simulink library "outp"  (Simulink 8.2)
settings: Solver=ode45  SolverMode=SingleTasking  StartTime=0.0  StopTime=10.0  RelTol=1e-3
undefined symbols (not defined in the file or in its folder): EPSILON, KOUTP_ACCSetSpeed_kph_defval, KOUTP_ACCSetSpeed_kph_maxval, KOUTP_ACCSetSpeed_kph_minval, KOUTP_ACCSetSpeed_kph_ovrdflg, KOUTP_ACCSetSpeed_kph_ovrdval, KOUTP_ACCSetSpeed_kph_srvcflg, KOUTP_ACCSetSpeed_kph_srvcval, KOUTP_ACCSetTimeGap_enum_defval, KOUTP_ACCSetTimeGap_enum_ovrdflg, KOUTP_ACCSetTimeGap_enum_ovrdval, KOUTP_ACCSetTimeGap_enum_srvcflg, KOUTP_ACCSetTimeGap_enum_srvcval, KOUTP_ACCSetTimeGapTmp_enum_defval, KOUTP_ACCSetTimeGapTmp_enum_ovrdflg, KOUTP_ACCSetTimeGapTmp_enum_ovrdval, KOUTP_ACCSetTimeGapTmp_enum_srvcflg, KOUTP_ACCSetTimeGapTmp_enum_srvcval, KOUTP_ACCWarningReq_flg_defval, KOUTP_ACCWarningReq_flg_ovrdflg, KOUTP_ACCWarningReq_flg_ovrdval, KOUTP_ACCWarningReq_flg_srvcflg, KOUTP_ACCWarningReq_flg_srvcval, KOUTP_ADAS1RollCnt_cnt_defval, KOUTP_ADAS1RollCnt_cnt_ovrdflg, KOUTP_ADAS1RollCnt_cnt_ovrdval, KOUTP_ADAS1RollCnt_cnt_srvcflg, KOUTP_ADAS1RollCnt_cnt_srvcval, KOUTP_ADAS2RollCnt_cnt_defval, KOUTP_ADAS2RollCnt_cnt_ovrdflg, KOUTP_ADAS2RollCnt_cnt_ovrdval, KOUTP_ADAS2RollCnt_cnt_srvcflg, KOUTP_ADAS2RollCnt_cnt_srvcval, KOUTP_ADAS3RollCnt_cnt_defval, KOUTP_ADAS3RollCnt_cnt_ovrdflg, KOUTP_ADAS3RollCnt_cnt_ovrdval, KOUTP_ADAS3RollCnt_cnt_srvcflg, KOUTP_ADAS3RollCnt_cnt_srvcval, KOUTP_ADASACCStatus_enum_defval, KOUTP_ADASACCStatus_enum_ovrdflg, KOUTP_ADASACCStatus_enum_ovrdval, KOUTP_ADASACCStatus_enum_srvcflg, KOUTP_ADASACCStatus_enum_srvcval, KOUTP_ADASFaultMode_enum_defval, KOUTP_ADASFaultMode_enum_ovrdflg, KOUTP_ADASFaultMode_enum_ovrdval, KOUTP_ADASFaultMode_enum_srvcflg, KOUTP_ADASFaultMode_enum_srvcval, KOUTP_ADASFunOffSoundReq_flg_defval, KOUTP_ADASFunOffSoundReq_flg_ovrdflg, KOUTP_ADASFunOffSoundReq_flg_ovrdval, KOUTP_ADASFunOffSoundReq_flg_srvcflg, KOUTP_ADASFunOffSoundReq_flg_srvcval, KOUTP_ADASFunOnSoundReq_flg_defval, KOUTP_ADASFunOnSoundReq_flg_ovrdflg, KOUTP_ADASFunOnSoundReq_flg_ovrdval, KOUTP_ADASFunOnSoundReq_flg_srvcflg, KOUTP_ADASFunOnSoundReq_flg_srvcval, KOUTP_ADASLFCStatus_enum_defval, KOUTP_ADASLFCStatus_enum_ovrdflg ... (+216)
libraries: outp x52, hcu_lib x8, simulink x3
(part 1 of 2)
settings Model: Creator=WX  LastModifiedBy=14014

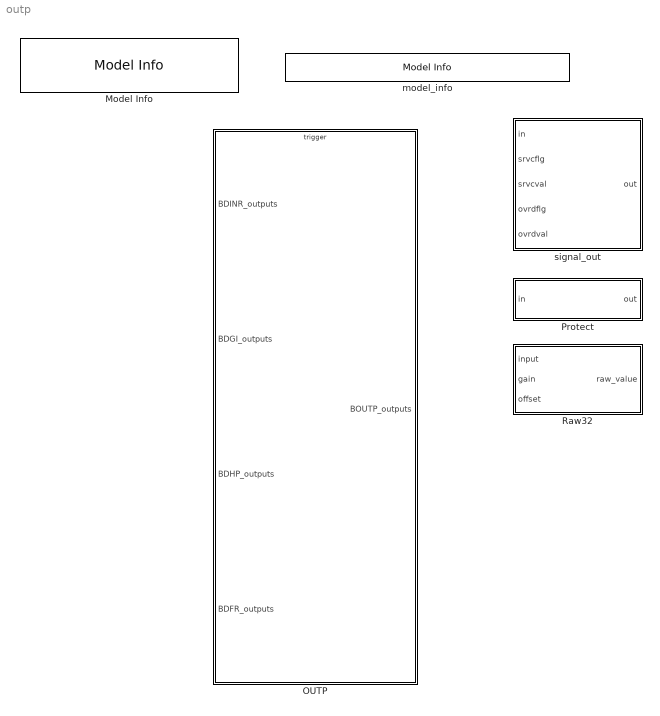
== system outp ==
  Model Info : simulink/Model-Wide Utilities/Model Info  InitialBlockCM=None  BlockCM=None  Frame=on  DisplayStringWithTags=|  HorizontalTextAlignment=Left  LeftAlignmentValue=0.02  SourceBlockDiagram=outp  TagMaxNumber=20
      | Model Version        : %<ModelVersion>
      | Creator                   : %<Creator>
      | Last Modified by    : %<LastModifiedBy>
  OUTP : Subsystem  TreatAsAtomicUnit=on
      settings: RTWSystemCode=Nonreusable function  RTWFcnNameOpts=Use subsystem name  RTWFileNameOpts=Use subsystem name
  Protect : Subsystem
  Raw32 : Subsystem
  model_info : simulink/Model-Wide Utilities/Model Info  InitialBlockCM=None  BlockCM=None  Frame=on  DisplayStringWithTags=$Id: hcu_lib.mdl 289 2016-04-11 06:01:08Z chimotsai $  HorizontalTextAlignment=Center  LeftAlignmentValue=0.5  SourceBlockDiagram=outp  TagMaxNumber=20
  signal_out : Subsystem

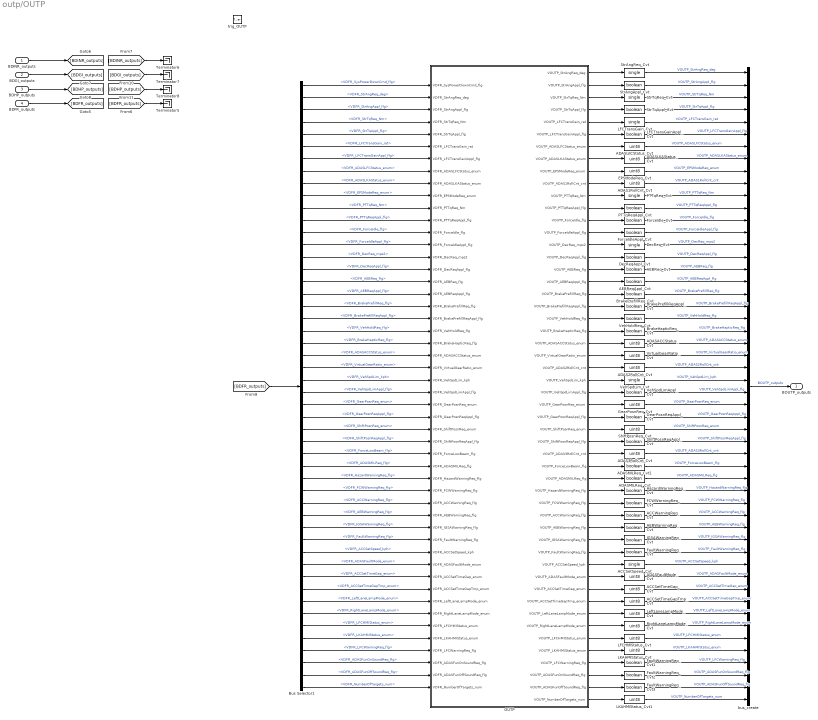
== system outp/OUTP ==
  BDINR_outputs : Inport  OutDataTypeStr=Bus: BDINR_outputs
  BDGI_outputs : Inport  Port=2  OutDataTypeStr=Bus: BDGI_outputs
  BDHP_outputs : Inport  Port=3  OutDataTypeStr=Bus: BDHP_outputs
  BDFR_outputs : Inport  Port=4  OutDataTypeStr=Bus: BDFR_outputs
  trig_OUTP : TriggerPort  TriggerType=function-call
  ACCSetSpeed_Cvt : DataTypeConversion  OutDataTypeStr=single  SaturateOnIntegerOverflow=on  RndMeth=Zero
  ACCSetTimeGapTmp_Cvt : DataTypeConversion  OutDataTypeStr=uint8  SaturateOnIntegerOverflow=on  RndMeth=Zero
  ACCSetTimeGap_Cvt : DataTypeConversion  OutDataTypeStr=uint8  SaturateOnIntegerOverflow=on  RndMeth=Zero
  ACCWarningReq_Cvt : DataTypeConversion  OutDataTypeStr=boolean  SaturateOnIntegerOverflow=on  RndMeth=Zero
  ADAS1RollCnt_Cvt : DataTypeConversion  OutDataTypeStr=uint8  SaturateOnIntegerOverflow=on  RndMeth=Zero
  ADAS2RollCnt_Cvt : DataTypeConversion  OutDataTypeStr=uint8  SaturateOnIntegerOverflow=on  RndMeth=Zero
  ADAS3RollCnt_Cvt : DataTypeConversion  OutDataTypeStr=uint8  SaturateOnIntegerOverflow=on  RndMeth=Zero
  ADASACCStatus_Cvt : DataTypeConversion  OutDataTypeStr=uint8  SaturateOnIntegerOverflow=on  RndMeth=Zero
  ADASFaultMode_Cvt : DataTypeConversion  OutDataTypeStr=uint8  SaturateOnIntegerOverflow=on  RndMeth=Zero
  ADASLFCStatus_Cvt : DataTypeConversion  OutDataTypeStr=uint8  SaturateOnIntegerOverflow=on  RndMeth=Zero
  ADASLKAStatus_Cvt : DataTypeConversion  OutDataTypeStr=uint8  SaturateOnIntegerOverflow=on  RndMeth=Zero
  ADASMILReq_Cvt : DataTypeConversion  OutDataTypeStr=boolean  SaturateOnIntegerOverflow=on  RndMeth=Zero
  ADASMILReq_Cvt1 : DataTypeConversion  OutDataTypeStr=boolean  SaturateOnIntegerOverflow=on  RndMeth=Zero
  AEBReqAppl_Cvt : DataTypeConversion  OutDataTypeStr=boolean  SaturateOnIntegerOverflow=on  RndMeth=Zero
  AEBReq_Cvt : DataTypeConversion  OutDataTypeStr=boolean  SaturateOnIntegerOverflow=on  RndMeth=Zero
  AEBWarningReq_Cvt : DataTypeConversion  OutDataTypeStr=boolean  SaturateOnIntegerOverflow=on  RndMeth=Zero
  BrakeHapticReq_Cvt : DataTypeConversion  OutDataTypeStr=boolean  SaturateOnIntegerOverflow=on  RndMeth=Zero
  BrakePrefillReqAppl_Cvt : DataTypeConversion  OutDataTypeStr=boolean  SaturateOnIntegerOverflow=on  RndMeth=Zero
  BrakePrefillReq_Cvt : DataTypeConversion  OutDataTypeStr=boolean  SaturateOnIntegerOverflow=on  RndMeth=Zero
  Bus Selector1 : BusSelector  OutputSignals=VDFR_SysPowerDownCmd_flg,VDFR_StrAngReq_deg,VDFR_StrAngAppl_flg,VDFR_StrTqReq_Nm,VDFR_StrTqAppl_flg,VDFR_LFCTransGain_rat,VDFR_LFCTransGainAppl_flg,VDFR_ADASLFCStatus_enum,VDFR_ADASLKAStatus_enum,VDFR_EPSModeReq_enum,VDFR_PTTqReq_Nm,VDFR_PTTqReqAppl_flg,VDFR_ForceIdle_flg,VDFR_ForceIdleAppl_flg,VDFR_DecReq_mps2,VDFR_DecReqAppl_flg,VDFR_AEBReq_flg,VDFR_AEBReqAppl_flg,VDFR_BrakePrefillReq_flg,VDFR_BrakePrefillReqAppl_flg,VDFR_VehHoldReq_flg,VDFR_BrakeHapticReq_flg,VDFR_ADASACCStatus_enum,VDFR_VirtualGearRatio_enum,VDFR_VehSpdLim_kph,VDFR_VehSpdLimAppl_flg,VDFR_GearPosnReq_enum,VDFR_GearPosnReqAppl_flg,VDFR_ShiftPosnReq_enum,VDFR_ShiftPosnReqAppl_flg,VDFR_ForceLowBeam_flg,VDFR_ADASMILReq_flg,VDFR_HazardWarningReq_flg,VDFR_FCWWarningReq_flg,VDFR_ACCWarningReq_flg,VDFR_AEBWarningReq_flg,VDFR_IGSAWarningReq_flg,VDFR_FaultWarningReq_flg,VDFR_ACCSetSpeed_kph,VDFR_ADASFaultMode_enum,VDFR_ACCSetTimeGap_enum,VDFR_ACCSetTimeGapTmp_enum,VDFR_LeftLaneLampMode_enum,VDFR_RightLaneLampMode_enum,VDFR_LFCHMIStatus_enum,VDFR_LKAHMIStatus_enum,VDFR_LFCWarningReq_flg,VDFR_ADASFunOnSoundReq_flg,VDFR_ADASFunOffSoundReq_flg,VDFR_NumberOfTargets_num
  DecReqAppl_Cvt : DataTypeConversion  OutDataTypeStr=boolean  SaturateOnIntegerOverflow=on  RndMeth=Zero
  DecReq_Cvt : DataTypeConversion  OutDataTypeStr=single  SaturateOnIntegerOverflow=on  RndMeth=Zero
  EPSModeReq_Cvt : DataTypeConversion  OutDataTypeStr=uint8  SaturateOnIntegerOverflow=on  RndMeth=Zero
  FCWWarningReq_Cvt : DataTypeConversion  OutDataTypeStr=boolean  SaturateOnIntegerOverflow=on  RndMeth=Zero
  FaultWarningReq_Cvt{,1..3} (4 alike) : DataTypeConversion  OutDataTypeStr=boolean  SaturateOnIntegerOverflow=on  RndMeth=Zero
  ForceIdleAppl_Cvt : DataTypeConversion  OutDataTypeStr=boolean  SaturateOnIntegerOverflow=on  RndMeth=Zero
  ForceIdle_Cvt : DataTypeConversion  OutDataTypeStr=boolean  SaturateOnIntegerOverflow=on  RndMeth=Zero
  GearPosnReqAppl_Cvt : DataTypeConversion  OutDataTypeStr=boolean  SaturateOnIntegerOverflow=on  RndMeth=Zero
  GearPosnReq_Cvt : DataTypeConversion  OutDataTypeStr=uint8  SaturateOnIntegerOverflow=on  RndMeth=Zero
  HazardWarningReq_Cvt : DataTypeConversion  OutDataTypeStr=boolean  SaturateOnIntegerOverflow=on  RndMeth=Zero
  IGSAWarningReq_Cvt : DataTypeConversion  OutDataTypeStr=boolean  SaturateOnIntegerOverflow=on  RndMeth=Zero
  LFCHMIStatus_Cvt : DataTypeConversion  OutDataTypeStr=uint8  SaturateOnIntegerOverflow=on  RndMeth=Zero
  LFCTransGainAppl_Cvt : DataTypeConversion  OutDataTypeStr=boolean  SaturateOnIntegerOverflow=on  RndMeth=Zero
  LFCTransGain_Cvt : DataTypeConversion  OutDataTypeStr=single  SaturateOnIntegerOverflow=on  RndMeth=Zero
  LKAHMIStatus_Cvt : DataTypeConversion  OutDataTypeStr=uint8  SaturateOnIntegerOverflow=on  RndMeth=Zero
  LKAHMIStatus_Cvt1 : DataTypeConversion  OutDataTypeStr=uint8  SaturateOnIntegerOverflow=on  RndMeth=Zero
  LeftLaneLampMode_Cvt : DataTypeConversion  OutDataTypeStr=uint8  SaturateOnIntegerOverflow=on  RndMeth=Zero
  OUTP : Subsystem
  PTTqReqAppl_Cvt : DataTypeConversion  OutDataTypeStr=boolean  SaturateOnIntegerOverflow=on  RndMeth=Zero
  PTTqReq_Cvt : DataTypeConversion  OutDataTypeStr=single  SaturateOnIntegerOverflow=on  RndMeth=Zero
  RightLaneLampMode_Cvt : DataTypeConversion  OutDataTypeStr=uint8  SaturateOnIntegerOverflow=on  RndMeth=Zero
  ShiftPosnReqAppl_Cvt : DataTypeConversion  OutDataTypeStr=boolean  SaturateOnIntegerOverflow=on  RndMeth=Zero
  ShiftPosnReq_Cvt : DataTypeConversion  OutDataTypeStr=uint8  SaturateOnIntegerOverflow=on  RndMeth=Zero
  StrAngAppl_Cvt : DataTypeConversion  OutDataTypeStr=boolean  SaturateOnIntegerOverflow=on  RndMeth=Zero
  StrAngReq_Cvt : DataTypeConversion  OutDataTypeStr=single  SaturateOnIntegerOverflow=on  RndMeth=Zero
  StrTqAppl_Cvt : DataTypeConversion  OutDataTypeStr=boolean  SaturateOnIntegerOverflow=on  RndMeth=Zero
  StrTqReq_Cvt : DataTypeConversion  OutDataTypeStr=single  SaturateOnIntegerOverflow=on  RndMeth=Zero
  Terminator{5..8} (4 alike) : Terminator
  VehHoldReq_Cvt : DataTypeConversion  OutDataTypeStr=boolean  SaturateOnIntegerOverflow=on  RndMeth=Zero
  VehSpdLimAppl_Cvt : DataTypeConversion  OutDataTypeStr=boolean  SaturateOnIntegerOverflow=on  RndMeth=Zero
  VehSpdLim_Cvt : DataTypeConversion  OutDataTypeStr=single  SaturateOnIntegerOverflow=on  RndMeth=Zero
  VirtualGearRatio_Cvt : DataTypeConversion  OutDataTypeStr=uint8  SaturateOnIntegerOverflow=on  RndMeth=Zero
  bus_create : BusCreator  Inputs=52  OutDataTypeStr=Bus: BOUTP_outputs
  BOUTP_outputs : Outport  OutDataTypeStr=Bus: BOUTP_outputs
  wires:
  [BDFR_outputs] -> Bus Selector1/1
  [BDFR_outputs] -> Terminator5/1
  BDFR_outputs/1 -> [BDFR_outputs]
  [BDINR_outputs] -> Terminator6/1
  BDINR_outputs/1 -> [BDINR_outputs]
  [BDGI_outputs] -> Terminator7/1
  BDGI_outputs/1 -> [BDGI_outputs]
  [BDHP_outputs] -> Terminator8/1
  BDHP_outputs/1 -> [BDHP_outputs]
  bus_create/1 -> BOUTP_outputs/1  "BOUTP_outputs"
  StrAngReq_Cvt/1 -> bus_create/1  "VOUTP_StrAngReq_deg"
  StrAngAppl_Cvt/1 -> bus_create/2  "VOUTP_StrAngAppl_flg"
  StrTqReq_Cvt/1 -> bus_create/3  "VOUTP_StrTqReq_Nm"
  StrTqAppl_Cvt/1 -> bus_create/4  "VOUTP_StrTqAppl_flg"
  LFCTransGain_Cvt/1 -> bus_create/5  "VOUTP_LFCTransGain_rat"
  LFCTransGainAppl_Cvt/1 -> bus_create/6  "VOUTP_LFCTransGainAppl_flg"
  ADASLFCStatus_Cvt/1 -> bus_create/7  "VOUTP_ADASLFCStatus_enum"
  ADASLKAStatus_Cvt/1 -> bus_create/8  "VOUTP_ADASLKAStatus_enum"
  EPSModeReq_Cvt/1 -> bus_create/9  "VOUTP_EPSModeReq_enum"
  ADAS1RollCnt_Cvt/1 -> bus_create/10  "VOUTP_ADAS1RollCnt_cnt"
  PTTqReq_Cvt/1 -> bus_create/11  "VOUTP_PTTqReq_Nm"
  ForceIdle_Cvt/1 -> bus_create/13  "VOUTP_ForceIdle_flg"
  PTTqReqAppl_Cvt/1 -> bus_create/12  "VOUTP_PTTqReqAppl_flg"
  DecReqAppl_Cvt/1 -> bus_create/16  "VOUTP_DecReqAppl_flg"
  ForceIdleAppl_Cvt/1 -> bus_create/14  "VOUTP_ForceIdleAppl_flg"
  DecReq_Cvt/1 -> bus_create/15  "VOUTP_DecReq_mps2"
  AEBReq_Cvt/1 -> bus_create/17  "VOUTP_AEBReq_flg"
  AEBReqAppl_Cvt/1 -> bus_create/18  "VOUTP_AEBReqAppl_flg"
  BrakePrefillReq_Cvt/1 -> bus_create/19  "VOUTP_BrakePrefillReq_flg"
  BrakePrefillReqAppl_Cvt/1 -> bus_create/20  "VOUTP_BrakePrefillReqAppl_flg"
  VehHoldReq_Cvt/1 -> bus_create/21  "VOUTP_VehHoldReq_flg"
  BrakeHapticReq_Cvt/1 -> bus_create/22  "VOUTP_BrakeHapticReq_flg"
  ADASACCStatus_Cvt/1 -> bus_create/23  "VOUTP_ADASACCStatus_enum"
  VirtualGearRatio_Cvt/1 -> bus_create/24  "VOUTP_VirtualGearRatio_enum"
  ADAS2RollCnt_Cvt/1 -> bus_create/25  "VOUTP_ADAS2RollCnt_cnt"
  VehSpdLim_Cvt/1 -> bus_create/26  "VOUTP_VehSpdLim_kph"
  VehSpdLimAppl_Cvt/1 -> bus_create/27  "VOUTP_VehSpdLimAppl_flg"
  GearPosnReq_Cvt/1 -> bus_create/28  "VOUTP_GearPosnReq_enum"
  GearPosnReqAppl_Cvt/1 -> bus_create/29  "VOUTP_GearPosnReqAppl_flg"
  ShiftPosnReq_Cvt/1 -> bus_create/30  "VOUTP_ShiftPosnReq_enum"
  ShiftPosnReqAppl_Cvt/1 -> bus_create/31  "VOUTP_ShiftPosnReqAppl_flg"
  ADAS3RollCnt_Cvt/1 -> bus_create/32  "VOUTP_ADAS3RollCnt_cnt"
  ADASMILReq_Cvt/1 -> bus_create/34  "VOUTP_ADASMILReq_flg"
  HazardWarningReq_Cvt/1 -> bus_create/35  "VOUTP_HazardWarningReq_flg"
  FCWWarningReq_Cvt/1 -> bus_create/36  "VOUTP_FCWWarningReq_flg"
  ACCWarningReq_Cvt/1 -> bus_create/37  "VOUTP_ACCWarningReq_flg"
  AEBWarningReq_Cvt/1 -> bus_create/38  "VOUTP_AEBWarningReq_flg"
  IGSAWarningReq_Cvt/1 -> bus_create/39  "VOUTP_IGSAWarningReq_flg"
  FaultWarningReq_Cvt/1 -> bus_create/40  "VOUTP_FaultWarningReq_flg"
  ACCSetSpeed_Cvt/1 -> bus_create/41  "VOUTP_ACCSetSpeed_kph"
  ADASFaultMode_Cvt/1 -> bus_create/42  "VOUTP_ADASFaultMode_enum"
  ACCSetTimeGap_Cvt/1 -> bus_create/43  "VOUTP_ACCSetTimeGap_enum"
  ACCSetTimeGapTmp_Cvt/1 -> bus_create/44  "VOUTP_ACCSetTimeGapTmp_enum"
  LeftLaneLampMode_Cvt/1 -> bus_create/45  "VOUTP_LeftLaneLampMode_enum"
  RightLaneLampMode_Cvt/1 -> bus_create/46  "VOUTP_RightLaneLampMode_enum"
  LFCHMIStatus_Cvt/1 -> bus_create/47  "VOUTP_LFCHMIStatus_enum"
  LKAHMIStatus_Cvt/1 -> bus_create/48  "VOUTP_LKAHMIStatus_enum"
  ADASMILReq_Cvt1/1 -> bus_create/33  "VOUTP_ForceLowBeam_flg"
  OUTP/30(VOUTP_ShiftPosnReq_enum) -> ShiftPosnReq_Cvt/1
  OUTP/14(VOUTP_ForceIdleAppl_flg) -> ForceIdleAppl_Cvt/1
  OUTP/4(VOUTP_StrTqAppl_flg) -> StrTqAppl_Cvt/1
  OUTP/13(VOUTP_ForceIdle_flg) -> ForceIdle_Cvt/1
  OUTP/29(VOUTP_GearPosnReqAppl_flg) -> GearPosnReqAppl_Cvt/1
  OUTP/27(VOUTP_VehSpdLimAppl_flg) -> VehSpdLimAppl_Cvt/1
  OUTP/2(VOUTP_StrAngAppl_flg) -> StrAngAppl_Cvt/1
  OUTP/26(VOUTP_VehSpdLim_kph) -> VehSpdLim_Cvt/1
  OUTP/6(VOUTP_LFCTransGainAppl_flg) -> LFCTransGainAppl_Cvt/1
  OUTP/10(VOUTP_ADAS1RollCnt_cnt) -> ADAS1RollCnt_Cvt/1
  OUTP/35(VOUTP_HazardWarningReq_flg) -> HazardWarningReq_Cvt/1
  OUTP/18(VOUTP_AEBReqAppl_flg) -> AEBReqAppl_Cvt/1
  OUTP/38(VOUTP_AEBWarningReq_flg) -> AEBWarningReq_Cvt/1
  OUTP/43(VOUTP_ACCSetTimeGap_enum) -> ACCSetTimeGap_Cvt/1
  OUTP/41(VOUTP_ACCSetSpeed_kph) -> ACCSetSpeed_Cvt/1
  OUTP/31(VOUTP_ShiftPosnReqAppl_flg) -> ShiftPosnReqAppl_Cvt/1
  OUTP/8(VOUTP_ADASLKAStatus_enum) -> ADASLKAStatus_Cvt/1
  OUTP/44(VOUTP_ACCSetTimeGapTmp_enum) -> ACCSetTimeGapTmp_Cvt/1
  OUTP/47(VOUTP_LFCHMIStatus_enum) -> LFCHMIStatus_Cvt/1
  OUTP/17(VOUTP_AEBReq_flg) -> AEBReq_Cvt/1
  OUTP/34(VOUTP_ADASMILReq_flg) -> ADASMILReq_Cvt/1
  OUTP/16(VOUTP_DecReqAppl_flg) -> DecReqAppl_Cvt/1
  OUTP/5(VOUTP_LFCTransGain_rat) -> LFCTransGain_Cvt/1
  OUTP/32(VOUTP_ADAS3RollCnt_cnt) -> ADAS3RollCnt_Cvt/1
  OUTP/12(VOUTP_PTTqReqAppl_flg) -> PTTqReqAppl_Cvt/1
  OUTP/9(VOUTP_EPSModeReq_enum) -> EPSModeReq_Cvt/1
  OUTP/7(VOUTP_ADASLFCStatus_enum) -> ADASLFCStatus_Cvt/1
  OUTP/42(VOUTP_ADASFaultMode_enum) -> ADASFaultMode_Cvt/1
  OUTP/11(VOUTP_PTTqReq_Nm) -> PTTqReq_Cvt/1
  OUTP/3(VOUTP_StrTqReq_Nm) -> StrTqReq_Cvt/1
  OUTP/40(VOUTP_FaultWarningReq_flg) -> FaultWarningReq_Cvt/1
  OUTP/25(VOUTP_ADAS2RollCnt_cnt) -> ADAS2RollCnt_Cvt/1
  OUTP/36(VOUTP_FCWWarningReq_flg) -> FCWWarningReq_Cvt/1
  OUTP/48(VOUTP_LKAHMIStatus_enum) -> LKAHMIStatus_Cvt/1
  OUTP/22(VOUTP_BrakeHapticReq_flg) -> BrakeHapticReq_Cvt/1
  OUTP/37(VOUTP_ACCWarningReq_flg) -> ACCWarningReq_Cvt/1
  OUTP/46(VOUTP_RightLaneLampMode_enum) -> RightLaneLampMode_Cvt/1
  OUTP/15(VOUTP_DecReq_mps2) -> DecReq_Cvt/1
  OUTP/23(VOUTP_ADASACCStatus_enum) -> ADASACCStatus_Cvt/1
  OUTP/45(VOUTP_LeftLaneLampMode_enum) -> LeftLaneLampMode_Cvt/1
  OUTP/28(VOUTP_GearPosnReq_enum) -> GearPosnReq_Cvt/1
  OUTP/20(VOUTP_BrakePrefillReqAppl_flg) -> BrakePrefillReqAppl_Cvt/1
  OUTP/39(VOUTP_IGSAWarningReq_flg) -> IGSAWarningReq_Cvt/1
  OUTP/19(VOUTP_BrakePrefillReq_flg) -> BrakePrefillReq_Cvt/1
  OUTP/21(VOUTP_VehHoldReq_flg) -> VehHoldReq_Cvt/1
  OUTP/1(VOUTP_StrAngReq_deg) -> StrAngReq_Cvt/1
  OUTP/24(VOUTP_VirtualGearRatio_enum) -> VirtualGearRatio_Cvt/1
  OUTP/33(VOUTP_ForceLowBeam_flg) -> ADASMILReq_Cvt1/1
  Bus Selector1/7 -> OUTP/7(VDFR_LFCTransGainAppl_flg)  "<VDFR_LFCTransGainAppl_flg>"
  Bus Selector1/8 -> OUTP/8(VDFR_ADASLFCStatus_enum)  "<VDFR_ADASLFCStatus_enum>"
  Bus Selector1/9 -> OUTP/9(VDFR_ADASLKAStatus_enum)  "<VDFR_ADASLKAStatus_enum>"
  Bus Selector1/10 -> OUTP/10(VDFR_EPSModeReq_enum)  "<VDFR_EPSModeReq_enum>"
  Bus Selector1/11 -> OUTP/11(VDFR_PTTqReq_Nm)  "<VDFR_PTTqReq_Nm>"
  Bus Selector1/12 -> OUTP/12(VDFR_PTTqReqAppl_flg)  "<VDFR_PTTqReqAppl_flg>"
  Bus Selector1/13 -> OUTP/13(VDFR_ForceIdle_flg)  "<VDFR_ForceIdle_flg>"
  Bus Selector1/14 -> OUTP/14(VDFR_ForceIdleAppl_flg)  "<VDFR_ForceIdleAppl_flg>"
  Bus Selector1/16 -> OUTP/16(VDFR_DecReqAppl_flg)  "<VDFR_DecReqAppl_flg>"
  Bus Selector1/15 -> OUTP/15(VDFR_DecReq_mps2)  "<VDFR_DecReq_mps2>"
  Bus Selector1/17 -> OUTP/17(VDFR_AEBReq_flg)  "<VDFR_AEBReq_flg>"
  Bus Selector1/18 -> OUTP/18(VDFR_AEBReqAppl_flg)  "<VDFR_AEBReqAppl_flg>"
  Bus Selector1/6 -> OUTP/6(VDFR_LFCTransGain_rat)  "<VDFR_LFCTransGain_rat>"
  Bus Selector1/5 -> OUTP/5(VDFR_StrTqAppl_flg)  "<VDFR_StrTqAppl_flg>"
  Bus Selector1/19 -> OUTP/19(VDFR_BrakePrefillReq_flg)  "<VDFR_BrakePrefillReq_flg>"
  Bus Selector1/1 -> OUTP/1(VDFR_SysPowerDownCmd_flg)  "<VDFR_SysPowerDownCmd_flg>"
  Bus Selector1/4 -> OUTP/4(VDFR_StrTqReq_Nm)  "<VDFR_StrTqReq_Nm>"
  Bus Selector1/3 -> OUTP/3(VDFR_StrAngAppl_flg)  "<VDFR_StrAngAppl_flg>"
  Bus Selector1/2 -> OUTP/2(VDFR_StrAngReq_deg)  "<VDFR_StrAngReq_deg>"
  Bus Selector1/21 -> OUTP/21(VDFR_VehHoldReq_flg)  "<VDFR_VehHoldReq_flg>"
  Bus Selector1/20 -> OUTP/20(VDFR_BrakePrefillReqAppl_flg)  "<VDFR_BrakePrefillReqAppl_flg>"
  Bus Selector1/22 -> OUTP/22(VDFR_BrakeHapticReq_flg)  "<VDFR_BrakeHapticReq_flg>"
  Bus Selector1/23 -> OUTP/23(VDFR_ADASACCStatus_enum)  "<VDFR_ADASACCStatus_enum>"
  Bus Selector1/35 -> OUTP/35(VDFR_ACCWarningReq_flg)  "<VDFR_ACCWarningReq_flg>"
  Bus Selector1/37 -> OUTP/37(VDFR_IGSAWarningReq_flg)  "<VDFR_IGSAWarningReq_flg>"
  Bus Selector1/28 -> OUTP/28(VDFR_GearPosnReqAppl_flg)  "<VDFR_GearPosnReqAppl_flg>"
  Bus Selector1/26 -> OUTP/26(VDFR_VehSpdLimAppl_flg)  "<VDFR_VehSpdLimAppl_flg>"
  Bus Selector1/31 -> OUTP/31(VDFR_ForceLowBeam_flg)  "<VDFR_ForceLowBeam_flg>"
  Bus Selector1/24 -> OUTP/24(VDFR_VirtualGearRatio_enum)  "<VDFR_VirtualGearRatio_enum>"
  Bus Selector1/33 -> OUTP/33(VDFR_HazardWarningReq_flg)  "<VDFR_HazardWarningReq_flg>"
  Bus Selector1/41 -> OUTP/41(VDFR_ACCSetTimeGap_enum)  "<VDFR_ACCSetTimeGap_enum>"
  Bus Selector1/34 -> OUTP/34(VDFR_FCWWarningReq_flg)  "<VDFR_FCWWarningReq_flg>"
  Bus Selector1/43 -> OUTP/43(VDFR_LeftLaneLampMode_enum)  "<VDFR_LeftLaneLampMode_enum>"
  Bus Selector1/30 -> OUTP/30(VDFR_ShiftPosnReqAppl_flg)  "<VDFR_ShiftPosnReqAppl_flg>"
  Bus Selector1/40 -> OUTP/40(VDFR_ADASFaultMode_enum)  "<VDFR_ADASFaultMode_enum>"
  Bus Selector1/38 -> OUTP/38(VDFR_FaultWarningReq_flg)  "<VDFR_FaultWarningReq_flg>"
  Bus Selector1/36 -> OUTP/36(VDFR_AEBWarningReq_flg)  "<VDFR_AEBWarningReq_flg>"
  Bus Selector1/29 -> OUTP/29(VDFR_ShiftPosnReq_enum)  "<VDFR_ShiftPosnReq_enum>"
  Bus Selector1/46 -> OUTP/46(VDFR_LKAHMIStatus_enum)  "<VDFR_LKAHMIStatus_enum>"
  Bus Selector1/27 -> OUTP/27(VDFR_GearPosnReq_enum)  "<VDFR_GearPosnReq_enum>"
  Bus Selector1/32 -> OUTP/32(VDFR_ADASMILReq_flg)  "<VDFR_ADASMILReq_flg>"
  Bus Selector1/45 -> OUTP/45(VDFR_LFCHMIStatus_enum)  "<VDFR_LFCHMIStatus_enum>"
  Bus Selector1/25 -> OUTP/25(VDFR_VehSpdLim_kph)  "<VDFR_VehSpdLim_kph>"
  Bus Selector1/44 -> OUTP/44(VDFR_RightLaneLampMode_enum)  "<VDFR_RightLaneLampMode_enum>"
  Bus Selector1/39 -> OUTP/39(VDFR_ACCSetSpeed_kph)  "<VDFR_ACCSetSpeed_kph>"
  Bus Selector1/42 -> OUTP/42(VDFR_ACCSetTimeGapTmp_enum)  "<VDFR_ACCSetTimeGapTmp_enum>"
  Bus Selector1/48 -> OUTP/48(VDFR_ADASFunOnSoundReq_flg)  "<VDFR_ADASFunOnSoundReq_flg>"
  Bus Selector1/47 -> OUTP/47(VDFR_LFCWarningReq_flg)  "<VDFR_LFCWarningReq_flg>"
  Bus Selector1/50 -> OUTP/50(VDFR_NumberOfTargets_num)  "<VDFR_NumberOfTargets_num>"
  Bus Selector1/49 -> OUTP/49(VDFR_ADASFunOffSoundReq_flg)  "<VDFR_ADASFunOffSoundReq_flg>"
  OUTP/49(VOUTP_LFCWarningReq_flg) -> FaultWarningReq_Cvt1/1
  OUTP/50(VOUTP_ADASFunOnSoundReq_flg) -> FaultWarningReq_Cvt2/1
  OUTP/51(VOUTP_ADASFunOffSoundReq_flg) -> FaultWarningReq_Cvt3/1
  OUTP/52(VOUTP_NumberOfTargets_num) -> LKAHMIStatus_Cvt1/1
  LKAHMIStatus_Cvt1/1 -> bus_create/52  "VOUTP_NumberOfTargets_num"
  FaultWarningReq_Cvt3/1 -> bus_create/51  "VOUTP_ADASFunOffSoundReq_flg"
  FaultWarningReq_Cvt1/1 -> bus_create/49  "VOUTP_LFCWarningReq_flg"
  FaultWarningReq_Cvt2/1 -> bus_create/50  "VOUTP_ADASFunOnSoundReq_flg"

== system outp/Protect ==
  in : Inport
  Bias : Bias  Bias=1
  Bitwise Operator : simulink/Logic and Bit Operations/Bitwise Operator  logicop=NOT  UseBitMask=off  BitMask=bin2dec('11011001')  BitMaskRealWorld=Stored Integer
  out : Outport
  wires:
  Bitwise Operator/1 -> Bias/1
  Bias/1 -> out/1
  in/1 -> Bitwise Operator/1

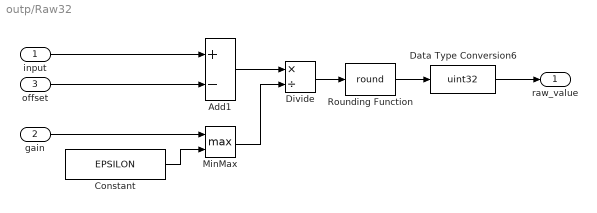
== system outp/Raw32 ==
  input : Inport
  gain : Inport  Port=2
  offset : Inport  Port=3
  Add1 : Sum  Inputs=+-
  Constant : Constant  Value=EPSILON
  Data Type Conversion6 : DataTypeConversion  OutDataTypeStr=uint32
  Divide : Product  Inputs=*/
  MinMax : MinMax  Function=max  Inputs=2
  Rounding Function : Rounding  Operator=round
  raw_value : Outport
  wires:
  Data Type Conversion6/1 -> raw_value/1
  Rounding Function/1 -> Data Type Conversion6/1
  input/1 -> Add1/1
  offset/1 -> Add1/2
  Add1/1 -> Divide/1
  Divide/1 -> Rounding Function/1
  gain/1 -> MinMax/1
  MinMax/1 -> Divide/2
  Constant/1 -> MinMax/2

== system outp/signal_out ==
  in : Inport
  srvcflg : Inport  Port=2
  srvcval : Inport  Port=3
  ovrdflg : Inport  Port=4
  ovrdval : Inport  Port=5
  Constant1 : Constant  Value=TRUE  OutDataTypeStr=Inherit: Inherit via back propagation
  Terminator13 : Terminator
  override signal : hcu_lib/override signal
  out : Outport
  wires:
  in/1 -> override signal/2
  override signal/1 -> out/1
  Constant1/1 -> override signal/1
  srvcflg/1 -> override signal/3
  srvcval/1 -> override signal/4
  ovrdflg/1 -> override signal/5
  ovrdval/1 -> override signal/6
  override signal/2 -> Terminator13/1

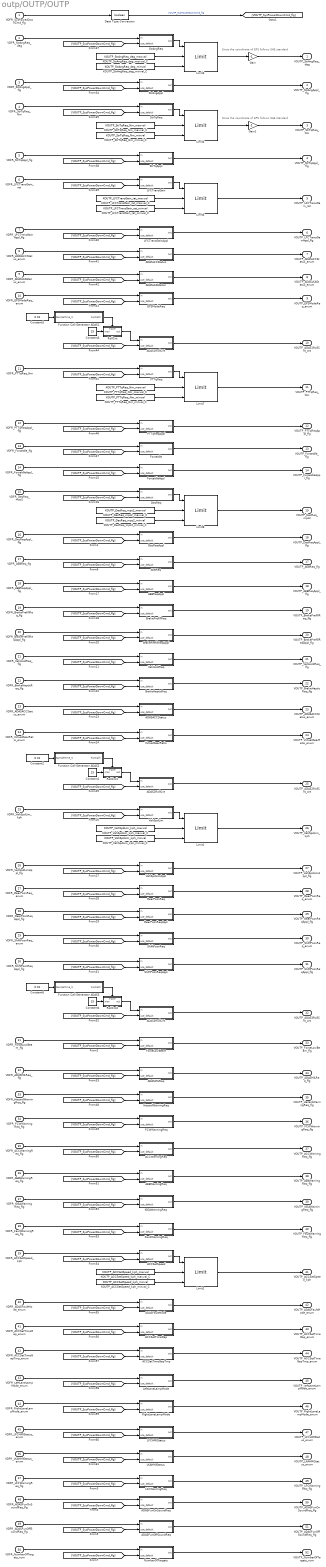
== system outp/OUTP/OUTP ==
  note: Since the coordinate of EPS follows SAE standard
  note: Since the coordinate of EPS follows SAE standard
  VDFR_SysPowerDownCmd_flg : Inport
  VDFR_StrAngReq_deg : Inport  Port=2
  VDFR_StrAngAppl_flg : Inport  Port=3
  VDFR_StrTqReq_Nm : Inport  Port=4
  VDFR_StrTqAppl_flg : Inport  Port=5
  VDFR_LFCTransGain_rat : Inport  Port=6
  VDFR_LFCTransGainAppl_flg : Inport  Port=7
  VDFR_ADASLFCStatus_enum : Inport  Port=8
  VDFR_ADASLKAStatus_enum : Inport  Port=9
  VDFR_EPSModeReq_enum : Inport  Port=10
  VDFR_PTTqReq_Nm : Inport  Port=11
  VDFR_PTTqReqAppl_flg : Inport  Port=12
  VDFR_ForceIdle_flg : Inport  Port=13
  VDFR_ForceIdleAppl_flg : Inport  Port=14
  VDFR_DecReq_mps2 : Inport  Port=15
  VDFR_DecReqAppl_flg : Inport  Port=16
  VDFR_AEBReq_flg : Inport  Port=17
  VDFR_AEBReqAppl_flg : Inport  Port=18
  VDFR_BrakePrefillReq_flg : Inport  Port=19
  VDFR_BrakePrefillReqAppl_flg : Inport  Port=20
  VDFR_VehHoldReq_flg : Inport  Port=21
  VDFR_BrakeHapticReq_flg : Inport  Port=22
  VDFR_ADASACCStatus_enum : Inport  Port=23
  VDFR_VirtualGearRatio_enum : Inport  Port=24
  VDFR_VehSpdLim_kph : Inport  Port=25
  VDFR_VehSpdLimAppl_flg : Inport  Port=26
  VDFR_GearPosnReq_enum : Inport  Port=27
  VDFR_GearPosnReqAppl_flg : Inport  Port=28
  VDFR_ShiftPosnReq_enum : Inport  Port=29
  VDFR_ShiftPosnReqAppl_flg : Inport  Port=30
  VDFR_ForceLowBeam_flg : Inport  Port=31
  VDFR_ADASMILReq_flg : Inport  Port=32
  VDFR_HazardWarningReq_flg : Inport  Port=33
  VDFR_FCWWarningReq_flg : Inport  Port=34
  VDFR_ACCWarningReq_flg : Inport  Port=35
  VDFR_AEBWarningReq_flg : Inport  Port=36
  VDFR_IGSAWarningReq_flg : Inport  Port=37
  VDFR_FaultWarningReq_flg : Inport  Port=38
  VDFR_ACCSetSpeed_kph : Inport  Port=39
  VDFR_ADASFaultMode_enum : Inport  Port=40
  VDFR_ACCSetTimeGap_enum : Inport  Port=41
  VDFR_ACCSetTimeGapTmp_enum : Inport  Port=42
  VDFR_LeftLaneLampMode_enum : Inport  Port=43
  VDFR_RightLaneLampMode_enum : Inport  Port=44
  VDFR_LFCHMIStatus_enum : Inport  Port=45
  VDFR_LKAHMIStatus_enum : Inport  Port=46
  VDFR_LFCWarningReq_flg : Inport  Port=47
  VDFR_ADASFunOnSoundReq_flg : Inport  Port=48
  VDFR_ADASFunOffSoundReq_flg : Inport  Port=49
  VDFR_NumberOfTargets_num : Inport  Port=50
  ACCSetSpeed : Subsystem
  ACCSetTimeGap : Subsystem
  ACCSetTimeGapTmp : Subsystem
  ACCWarningReq : Subsystem
  ADAS1RollCnt : Subsystem
  ADAS2RollCnt : Subsystem
  ADAS3RollCnt : Subsystem
  ADASACCStatus : Subsystem
  ADASFaultMode : Subsystem
  ADASFunOffSoundReq : Subsystem
  ADASFunOnSoundReq : Subsystem
  ADASLFCStatus : Subsystem
  ADASLKAStatus : Subsystem
  ADASMILReq : Subsystem
  AEBReq : Subsystem
  AEBReqAppl : Subsystem
  AEBWarningReq : Subsystem
  BrakeHapticReq : Subsystem
  BrakePrefillReq : Subsystem
  BrakePrefillReqAppl : Subsystem
  Constant1 : Constant  Value=15  OutDataTypeStr=uint8
  Constant2 : Constant  Value=0.01
  Constant3 : Constant  Value=15  OutDataTypeStr=uint8
  Constant4 : Constant  Value=15  OutDataTypeStr=uint8
  Constant5 : Constant  Value=0.01
  Constant6 : Constant  Value=0.01
  Data Type Conversion : DataTypeConversion  OutDataTypeStr=boolean
  DecReq : Subsystem
  DecReqAppl : Subsystem
  EPSModeReq : Subsystem
  FCWWarningReq : Subsystem
  FaultWarningReq : Subsystem
  ForceIdle : Subsystem
  ForceIdleAppl : Subsystem
  ForceLowBeam : Subsystem
  Function Call Generator ADAS1 : Stateflow chart  TreatAsAtomicUnit=on
  Function Call Generator ADAS2 : Stateflow chart  TreatAsAtomicUnit=on
  Function Call Generator ADAS3 : Stateflow chart  TreatAsAtomicUnit=on
  Gain : Gain  Gain=-1
  Gain1 : Gain  Gain=-1
  GearPosnReq : Subsystem
  GearPosnReqAppl : Subsystem
  HazardWarningReq : Subsystem
  IGSAWarningReq : Subsystem
  KOUTP_ACCSetSpeed_kph_maxval_C : Constant  Value=KOUTP_ACCSetSpeed_kph_maxval
  KOUTP_ACCSetSpeed_kph_minval_C : Constant  Value=KOUTP_ACCSetSpeed_kph_minval
  KOUTP_DecReq_mps2_maxval_C : Constant  Value=KOUTP_DecReq_mps2_maxval
  KOUTP_DecReq_mps2_minval_C : Constant  Value=KOUTP_DecReq_mps2_minval
  KOUTP_LFCTransGain_rat_maxval_C : Constant  Value=KOUTP_LFCTransGain_rat_maxval
  KOUTP_LFCTransGain_rat_minval_C : Constant  Value=KOUTP_LFCTransGain_rat_minval
  KOUTP_PTTqReq_Nm_maxval_C : Constant  Value=KOUTP_PTTqReq_Nm_maxval
  KOUTP_PTTqReq_Nm_minval_C : Constant  Value=KOUTP_PTTqReq_Nm_minval
  KOUTP_StrAngReq_deg_maxval_C : Constant  Value=KOUTP_StrAngReq_deg_maxval
  KOUTP_StrAngReq_deg_minval_C : Constant  Value=KOUTP_StrAngReq_deg_minval
  KOUTP_StrTqReq_Nm_maxval_C : Constant  Value=KOUTP_StrTqReq_Nm_maxval
  KOUTP_StrTqReq_Nm_minval_C : Constant  Value=KOUTP_StrTqReq_Nm_minval
  KOUTP_VehSpdLim_kph_maxval_C : Constant  Value=KOUTP_VehSpdLim_kph_maxval
  KOUTP_VehSpdLim_kph_minval_C : Constant  Value=KOUTP_VehSpdLim_kph_minval
  LFCHMIStatus : Subsystem
  LFCTransGain : Subsystem
  LFCTransGainAppl : Subsystem
  LFCWarningReq : Subsystem
  LKAHMIStatus : Subsystem
  LeftLaneLampMode : Subsystem
  Limit{1..4,6..8} (7 alike) : hcu_lib/Limit  SystemSampleTime=-1
  NumberOfTargets : Subsystem
  PTTqReq : Subsystem
  PTTqReqAppl : Subsystem
  RightLaneLampMode : Subsystem
  RollCnt : Subsystem
  RollCnt1 : Subsystem
  RollCnt2 : Subsystem
  ShiftPosnReq : Subsystem
  ShiftPosnReqAppl : Subsystem
  StrAngAppl : Subsystem
  StrAngReq : Subsystem
  StrTqAppl : Subsystem
  StrTqReq : Subsystem
  VehHoldReq : Subsystem
  VehSpdLim : Subsystem
  VehSpdLimAppl : Subsystem
  VirtualGearRatio : Subsystem
  VOUTP_StrAngReq_deg : Outport
  VOUTP_StrAngAppl_flg : Outport  Port=2
  VOUTP_StrTqReq_Nm : Outport  Port=3
  VOUTP_StrTqAppl_flg : Outport  Port=4
  VOUTP_LFCTransGain_rat : Outport  Port=5
  VOUTP_LFCTransGainAppl_flg : Outport  Port=6
  VOUTP_ADASLFCStatus_enum : Outport  Port=7
  VOUTP_ADASLKAStatus_enum : Outport  Port=8
  VOUTP_EPSModeReq_enum : Outport  Port=9
  VOUTP_ADAS1RollCnt_cnt : Outport  Port=10
  VOUTP_PTTqReq_Nm : Outport  Port=11
  VOUTP_PTTqReqAppl_flg : Outport  Port=12
  VOUTP_ForceIdle_flg : Outport  Port=13
  VOUTP_ForceIdleAppl_flg : Outport  Port=14
  VOUTP_DecReq_mps2 : Outport  Port=15
  VOUTP_DecReqAppl_flg : Outport  Port=16
  VOUTP_AEBReq_flg : Outport  Port=17
  VOUTP_AEBReqAppl_flg : Outport  Port=18
  VOUTP_BrakePrefillReq_flg : Outport  Port=19
  VOUTP_BrakePrefillReqAppl_flg : Outport  Port=20
  VOUTP_VehHoldReq_flg : Outport  Port=21
  VOUTP_BrakeHapticReq_flg : Outport  Port=22
  VOUTP_ADASACCStatus_enum : Outport  Port=23
  VOUTP_VirtualGearRatio_enum : Outport  Port=24
  VOUTP_ADAS2RollCnt_cnt : Outport  Port=25
  VOUTP_VehSpdLim_kph : Outport  Port=26
  VOUTP_VehSpdLimAppl_flg : Outport  Port=27
  VOUTP_GearPosnReq_enum : Outport  Port=28
  VOUTP_GearPosnReqAppl_flg : Outport  Port=29
  VOUTP_ShiftPosnReq_enum : Outport  Port=30
  VOUTP_ShiftPosnReqAppl_flg : Outport  Port=31
  VOUTP_ADAS3RollCnt_cnt : Outport  Port=32
  VOUTP_ForceLowBeam_flg : Outport  Port=33
  VOUTP_ADASMILReq_flg : Outport  Port=34
  VOUTP_HazardWarningReq_flg : Outport  Port=35
  VOUTP_FCWWarningReq_flg : Outport  Port=36
  VOUTP_ACCWarningReq_flg : Outport  Port=37
  VOUTP_AEBWarningReq_flg : Outport  Port=38
  VOUTP_IGSAWarningReq_flg : Outport  Port=39
  VOUTP_FaultWarningReq_flg : Outport  Port=40
  VOUTP_ACCSetSpeed_kph : Outport  Port=41
  VOUTP_ADASFaultMode_enum : Outport  Port=42
  VOUTP_ACCSetTimeGap_enum : Outport  Port=43
  VOUTP_ACCSetTimeGapTmp_enum : Outport  Port=44
  VOUTP_LeftLaneLampMode_enum : Outport  Port=45
  VOUTP_RightLaneLampMode_enum : Outport  Port=46
  VOUTP_LFCHMIStatus_enum : Outport  Port=47
  VOUTP_LKAHMIStatus_enum : Outport  Port=48
  VOUTP_LFCWarningReq_flg : Outport  Port=49
  VOUTP_ADASFunOnSoundReq_flg : Outport  Port=50
  VOUTP_ADASFunOffSoundReq_flg : Outport  Port=51
  VOUTP_NumberOfTargets_num : Outport  Port=52
  wires:
  VDFR_SysPowerDownCmd_flg/1 -> Data Type Conversion/1
  StrAngAppl/1(out) -> VOUTP_StrAngAppl_flg/1
  VDFR_StrAngAppl_flg/1 -> StrAngAppl/1(in)
  Limit3/1 -> Gain/1
  VDFR_StrAngReq_deg/1 -> StrAngReq/1(in)
  KOUTP_StrAngReq_deg_maxval_C/1 -> Limit3/2
  KOUTP_StrAngReq_deg_minval_C/1 -> Limit3/3
  [VOUTP_SysPowerDownCmd_flg] -> StrAngReq/2(use_default)
  StrAngReq/1(out) -> Limit3/1
  Data Type Conversion/1 -> [VOUTP_SysPowerDownCmd_flg]  "VOUTP_SysPowerDownCmd_flg"
  [VOUTP_SysPowerDownCmd_flg] -> StrAngAppl/2(use_default)
  Limit4/1 -> Gain1/1
  VDFR_StrTqReq_Nm/1 -> StrTqReq/1(in)
  KOUTP_StrTqReq_Nm_maxval_C/1 -> Limit4/2
  KOUTP_StrTqReq_Nm_minval_C/1 -> Limit4/3
  [VOUTP_SysPowerDownCmd_flg] -> StrTqReq/2(use_default)
  StrTqReq/1(out) -> Limit4/1
  StrTqAppl/1(out) -> VOUTP_StrTqAppl_flg/1
  VDFR_StrTqAppl_flg/1 -> StrTqAppl/1(in)
  [VOUTP_SysPowerDownCmd_flg] -> StrTqAppl/2(use_default)
  Limit6/1 -> VOUTP_LFCTransGain_rat/1
  VDFR_LFCTransGain_rat/1 -> LFCTransGain/1(in)
  KOUTP_LFCTransGain_rat_maxval_C/1 -> Limit6/2
  KOUTP_LFCTransGain_rat_minval_C/1 -> Limit6/3
  [VOUTP_SysPowerDownCmd_flg] -> LFCTransGain/2(use_default)
  LFCTransGain/1(out) -> Limit6/1
  LFCTransGainAppl/1(out) -> VOUTP_LFCTransGainAppl_flg/1
  VDFR_LFCTransGainAppl_flg/1 -> LFCTransGainAppl/1(in)
  [VOUTP_SysPowerDownCmd_flg] -> LFCTransGainAppl/2(use_default)
  ADASLFCStatus/1(out) -> VOUTP_ADASLFCStatus_enum/1
  VDFR_ADASLFCStatus_enum/1 -> ADASLFCStatus/1(in)
  [VOUTP_SysPowerDownCmd_flg] -> ADASLFCStatus/2(use_default)
  ADASLKAStatus/1(out) -> VOUTP_ADASLKAStatus_enum/1
  VDFR_ADASLKAStatus_enum/1 -> ADASLKAStatus/1(in)
  [VOUTP_SysPowerDownCmd_flg] -> ADASLKAStatus/2(use_default)
  EPSModeReq/1(out) -> VOUTP_EPSModeReq_enum/1
  VDFR_EPSModeReq_enum/1 -> EPSModeReq/1(in)
  [VOUTP_SysPowerDownCmd_flg] -> EPSModeReq/2(use_default)
  ADAS1RollCnt/1(out) -> VOUTP_ADAS1RollCnt_cnt/1
  [VOUTP_SysPowerDownCmd_flg] -> ADAS1RollCnt/2(use_default)
  Constant3/1 -> RollCnt/1(max)
  Constant5/1 -> Function Call Generator ADAS1/1(SampleTime_S)
  Function Call Generator ADAS1/1(FunCall()) -> RollCnt/Trigger
  RollCnt/1(out) -> ADAS1RollCnt/1(in)
  Limit7/1 -> VOUTP_PTTqReq_Nm/1
  VDFR_PTTqReq_Nm/1 -> PTTqReq/1(in)
  KOUTP_PTTqReq_Nm_maxval_C/1 -> Limit7/2
  KOUTP_PTTqReq_Nm_minval_C/1 -> Limit7/3
  [VOUTP_SysPowerDownCmd_flg] -> PTTqReq/2(use_default)
  PTTqReq/1(out) -> Limit7/1
  PTTqReqAppl/1(out) -> VOUTP_PTTqReqAppl_flg/1
  VDFR_PTTqReqAppl_flg/1 -> PTTqReqAppl/1(in)
  [VOUTP_SysPowerDownCmd_flg] -> PTTqReqAppl/2(use_default)
  ForceIdle/1(out) -> VOUTP_ForceIdle_flg/1
  VDFR_ForceIdle_flg/1 -> ForceIdle/1(in)
  [VOUTP_SysPowerDownCmd_flg] -> ForceIdle/2(use_default)
  ForceIdleAppl/1(out) -> VOUTP_ForceIdleAppl_flg/1
  VDFR_ForceIdleAppl_flg/1 -> ForceIdleAppl/1(in)
  [VOUTP_SysPowerDownCmd_flg] -> ForceIdleAppl/2(use_default)
  Limit8/1 -> VOUTP_DecReq_mps2/1
  VDFR_DecReq_mps2/1 -> DecReq/1(in)
  KOUTP_DecReq_mps2_maxval_C/1 -> Limit8/2
  KOUTP_DecReq_mps2_minval_C/1 -> Limit8/3
  [VOUTP_SysPowerDownCmd_flg] -> DecReq/2(use_default)
  DecReq/1(out) -> Limit8/1
  DecReqAppl/1(out) -> VOUTP_DecReqAppl_flg/1
  VDFR_DecReqAppl_flg/1 -> DecReqAppl/1(in)
  [VOUTP_SysPowerDownCmd_flg] -> DecReqAppl/2(use_default)
  AEBReq/1(out) -> VOUTP_AEBReq_flg/1
  VDFR_AEBReq_flg/1 -> AEBReq/1(in)
  [VOUTP_SysPowerDownCmd_flg] -> AEBReq/2(use_default)
  AEBReqAppl/1(out) -> VOUTP_AEBReqAppl_flg/1
  VDFR_AEBReqAppl_flg/1 -> AEBReqAppl/1(in)
  [VOUTP_SysPowerDownCmd_flg] -> AEBReqAppl/2(use_default)
  BrakePrefillReq/1(out) -> VOUTP_BrakePrefillReq_flg/1
  VDFR_BrakePrefillReq_flg/1 -> BrakePrefillReq/1(in)
  [VOUTP_SysPowerDownCmd_flg] -> BrakePrefillReq/2(use_default)
  BrakePrefillReqAppl/1(out) -> VOUTP_BrakePrefillReqAppl_flg/1
  VDFR_BrakePrefillReqAppl_flg/1 -> BrakePrefillReqAppl/1(in)
  [VOUTP_SysPowerDownCmd_flg] -> BrakePrefillReqAppl/2(use_default)
  VehHoldReq/1(out) -> VOUTP_VehHoldReq_flg/1
  VDFR_VehHoldReq_flg/1 -> VehHoldReq/1(in)
  [VOUTP_SysPowerDownCmd_flg] -> VehHoldReq/2(use_default)
  BrakeHapticReq/1(out) -> VOUTP_BrakeHapticReq_flg/1
  VDFR_BrakeHapticReq_flg/1 -> BrakeHapticReq/1(in)
  [VOUTP_SysPowerDownCmd_flg] -> BrakeHapticReq/2(use_default)
  ADASACCStatus/1(out) -> VOUTP_ADASACCStatus_enum/1
  VDFR_ADASACCStatus_enum/1 -> ADASACCStatus/1(in)
  [VOUTP_SysPowerDownCmd_flg] -> ADASACCStatus/2(use_default)
  VirtualGearRatio/1(out) -> VOUTP_VirtualGearRatio_enum/1
  VDFR_VirtualGearRatio_enum/1 -> VirtualGearRatio/1(in)
  [VOUTP_SysPowerDownCmd_flg] -> VirtualGearRatio/2(use_default)
  ADAS2RollCnt/1(out) -> VOUTP_ADAS2RollCnt_cnt/1
  [VOUTP_SysPowerDownCmd_flg] -> ADAS2RollCnt/2(use_default)
  Constant1/1 -> RollCnt1/1(max)
  Constant2/1 -> Function Call Generator ADAS2/1(SampleTime_S)
  Function Call Generator ADAS2/1(FunCall()) -> RollCnt1/Trigger
  RollCnt1/1(out) -> ADAS2RollCnt/1(in)
  Limit1/1 -> VOUTP_VehSpdLim_kph/1
  VDFR_VehSpdLim_kph/1 -> VehSpdLim/1(in)
  KOUTP_VehSpdLim_kph_maxval_C/1 -> Limit1/2
  KOUTP_VehSpdLim_kph_minval_C/1 -> Limit1/3
  [VOUTP_SysPowerDownCmd_flg] -> VehSpdLim/2(use_default)
  VehSpdLim/1(out) -> Limit1/1
  VehSpdLimAppl/1(out) -> VOUTP_VehSpdLimAppl_flg/1
  VDFR_VehSpdLimAppl_flg/1 -> VehSpdLimAppl/1(in)
  [VOUTP_SysPowerDownCmd_flg] -> VehSpdLimAppl/2(use_default)
  GearPosnReq/1(out) -> VOUTP_GearPosnReq_enum/1
  VDFR_GearPosnReq_enum/1 -> GearPosnReq/1(in)
  [VOUTP_SysPowerDownCmd_flg] -> GearPosnReq/2(use_default)
  GearPosnReqAppl/1(out) -> VOUTP_GearPosnReqAppl_flg/1
  VDFR_GearPosnReqAppl_flg/1 -> GearPosnReqAppl/1(in)
  [VOUTP_SysPowerDownCmd_flg] -> GearPosnReqAppl/2(use_default)
  ShiftPosnReq/1(out) -> VOUTP_ShiftPosnReq_enum/1
  VDFR_ShiftPosnReq_enum/1 -> ShiftPosnReq/1(in)
  [VOUTP_SysPowerDownCmd_flg] -> ShiftPosnReq/2(use_default)
  ShiftPosnReqAppl/1(out) -> VOUTP_ShiftPosnReqAppl_flg/1
  VDFR_ShiftPosnReqAppl_flg/1 -> ShiftPosnReqAppl/1(in)
  [VOUTP_SysPowerDownCmd_flg] -> ShiftPosnReqAppl/2(use_default)
  ADAS3RollCnt/1(out) -> VOUTP_ADAS3RollCnt_cnt/1
  [VOUTP_SysPowerDownCmd_flg] -> ADAS3RollCnt/2(use_default)
  Constant4/1 -> RollCnt2/1(max)
  Constant6/1 -> Function Call Generator ADAS3/1(SampleTime_S)
  Function Call Generator ADAS3/1(FunCall()) -> RollCnt2/Trigger
  RollCnt2/1(out) -> ADAS3RollCnt/1(in)
  ADASMILReq/1(out) -> VOUTP_ADASMILReq_flg/1
  VDFR_ADASMILReq_flg/1 -> ADASMILReq/1(in)
  [VOUTP_SysPowerDownCmd_flg] -> ADASMILReq/2(use_default)
  HazardWarningReq/1(out) -> VOUTP_HazardWarningReq_flg/1
  VDFR_HazardWarningReq_flg/1 -> HazardWarningReq/1(in)
  [VOUTP_SysPowerDownCmd_flg] -> HazardWarningReq/2(use_default)
  FCWWarningReq/1(out) -> VOUTP_FCWWarningReq_flg/1
  VDFR_FCWWarningReq_flg/1 -> FCWWarningReq/1(in)
  [VOUTP_SysPowerDownCmd_flg] -> FCWWarningReq/2(use_default)
  ACCWarningReq/1(out) -> VOUTP_ACCWarningReq_flg/1
  VDFR_ACCWarningReq_flg/1 -> ACCWarningReq/1(in)
  [VOUTP_SysPowerDownCmd_flg] -> ACCWarningReq/2(use_default)
  AEBWarningReq/1(out) -> VOUTP_AEBWarningReq_flg/1
  VDFR_AEBWarningReq_flg/1 -> AEBWarningReq/1(in)
  [VOUTP_SysPowerDownCmd_flg] -> AEBWarningReq/2(use_default)
  IGSAWarningReq/1(out) -> VOUTP_IGSAWarningReq_flg/1
  VDFR_IGSAWarningReq_flg/1 -> IGSAWarningReq/1(in)
  [VOUTP_SysPowerDownCmd_flg] -> IGSAWarningReq/2(use_default)
  FaultWarningReq/1(out) -> VOUTP_FaultWarningReq_flg/1
  VDFR_FaultWarningReq_flg/1 -> FaultWarningReq/1(in)
  [VOUTP_SysPowerDownCmd_flg] -> FaultWarningReq/2(use_default)
  Limit2/1 -> VOUTP_ACCSetSpeed_kph/1
  VDFR_ACCSetSpeed_kph/1 -> ACCSetSpeed/1(in)
  KOUTP_ACCSetSpeed_kph_maxval_C/1 -> Limit2/2
  KOUTP_ACCSetSpeed_kph_minval_C/1 -> Limit2/3
  [VOUTP_SysPowerDownCmd_flg] -> ACCSetSpeed/2(use_default)
  ACCSetSpeed/1(out) -> Limit2/1
  ADASFaultMode/1(out) -> VOUTP_ADASFaultMode_enum/1
  VDFR_ADASFaultMode_enum/1 -> ADASFaultMode/1(in)
  [VOUTP_SysPowerDownCmd_flg] -> ADASFaultMode/2(use_default)
  ACCSetTimeGap/1(out) -> VOUTP_ACCSetTimeGap_enum/1
  VDFR_ACCSetTimeGap_enum/1 -> ACCSetTimeGap/1(in)
  [VOUTP_SysPowerDownCmd_flg] -> ACCSetTimeGap/2(use_default)
  ACCSetTimeGapTmp/1(out) -> VOUTP_ACCSetTimeGapTmp_enum/1
  VDFR_ACCSetTimeGapTmp_enum/1 -> ACCSetTimeGapTmp/1(in)
  [VOUTP_SysPowerDownCmd_flg] -> ACCSetTimeGapTmp/2(use_default)
  LeftLaneLampMode/1(out) -> VOUTP_LeftLaneLampMode_enum/1
  VDFR_LeftLaneLampMode_enum/1 -> LeftLaneLampMode/1(in)
  [VOUTP_SysPowerDownCmd_flg] -> LeftLaneLampMode/2(use_default)
  RightLaneLampMode/1(out) -> VOUTP_RightLaneLampMode_enum/1
  VDFR_RightLaneLampMode_enum/1 -> RightLaneLampMode/1(in)
  [VOUTP_SysPowerDownCmd_flg] -> RightLaneLampMode/2(use_default)
  LFCHMIStatus/1(out) -> VOUTP_LFCHMIStatus_enum/1
  VDFR_LFCHMIStatus_enum/1 -> LFCHMIStatus/1(in)
  [VOUTP_SysPowerDownCmd_flg] -> LFCHMIStatus/2(use_default)
  LKAHMIStatus/1(out) -> VOUTP_LKAHMIStatus_enum/1
  VDFR_LKAHMIStatus_enum/1 -> LKAHMIStatus/1(in)
  [VOUTP_SysPowerDownCmd_flg] -> LKAHMIStatus/2(use_default)
  ForceLowBeam/1(out) -> VOUTP_ForceLowBeam_flg/1
  VDFR_ForceLowBeam_flg/1 -> ForceLowBeam/1(in)
  [VOUTP_SysPowerDownCmd_flg] -> ForceLowBeam/2(use_default)
  Gain/1 -> VOUTP_StrAngReq_deg/1
  Gain1/1 -> VOUTP_StrTqReq_Nm/1
  LFCWarningReq/1(out) -> VOUTP_LFCWarningReq_flg/1
  VDFR_LFCWarningReq_flg/1 -> LFCWarningReq/1(in)
  [VOUTP_SysPowerDownCmd_flg] -> LFCWarningReq/2(use_default)
  ADASFunOnSoundReq/1(out) -> VOUTP_ADASFunOnSoundReq_flg/1
  VDFR_ADASFunOnSoundReq_flg/1 -> ADASFunOnSoundReq/1(in)
  [VOUTP_SysPowerDownCmd_flg] -> ADASFunOnSoundReq/2(use_default)
  ADASFunOffSoundReq/1(out) -> VOUTP_ADASFunOffSoundReq_flg/1
  VDFR_ADASFunOffSoundReq_flg/1 -> ADASFunOffSoundReq/1(in)
  [VOUTP_SysPowerDownCmd_flg] -> ADASFunOffSoundReq/2(use_default)
  NumberOfTargets/1(out) -> VOUTP_NumberOfTargets_num/1
  VDFR_NumberOfTargets_num/1 -> NumberOfTargets/1(in)
  [VOUTP_SysPowerDownCmd_flg] -> NumberOfTargets/2(use_default)

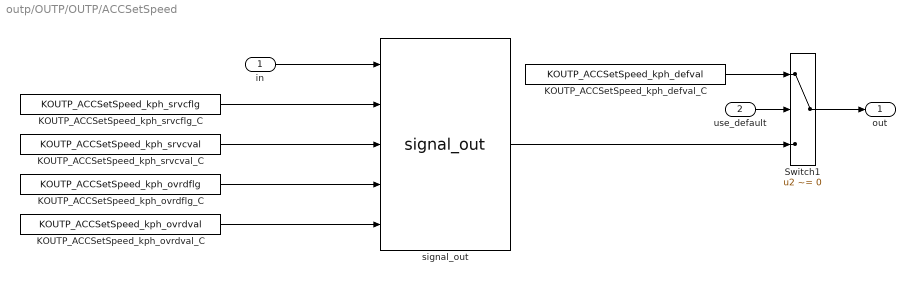
== system outp/OUTP/OUTP/ACCSetSpeed ==
  in : Inport
  use_default : Inport  Port=2
  KOUTP_ACCSetSpeed_kph_defval_C : Constant  Value=KOUTP_ACCSetSpeed_kph_defval
  KOUTP_ACCSetSpeed_kph_ovrdflg_C : Constant  Value=KOUTP_ACCSetSpeed_kph_ovrdflg
  KOUTP_ACCSetSpeed_kph_ovrdval_C : Constant  Value=KOUTP_ACCSetSpeed_kph_ovrdval
  KOUTP_ACCSetSpeed_kph_srvcflg_C : Constant  Value=KOUTP_ACCSetSpeed_kph_srvcflg
  KOUTP_ACCSetSpeed_kph_srvcval_C : Constant  Value=KOUTP_ACCSetSpeed_kph_srvcval
  Switch1 : Switch  Criteria=u2 ~= 0  Threshold=0.5
  signal_out : outp/signal_out
  out : Outport
  wires:
  in/1 -> signal_out/1
  signal_out/1 -> Switch1/3
  use_default/1 -> Switch1/2
  Switch1/1 -> out/1
  KOUTP_ACCSetSpeed_kph_srvcflg_C/1 -> signal_out/2
  KOUTP_ACCSetSpeed_kph_srvcval_C/1 -> signal_out/3
  KOUTP_ACCSetSpeed_kph_ovrdflg_C/1 -> signal_out/4
  KOUTP_ACCSetSpeed_kph_ovrdval_C/1 -> signal_out/5
  KOUTP_ACCSetSpeed_kph_defval_C/1 -> Switch1/1

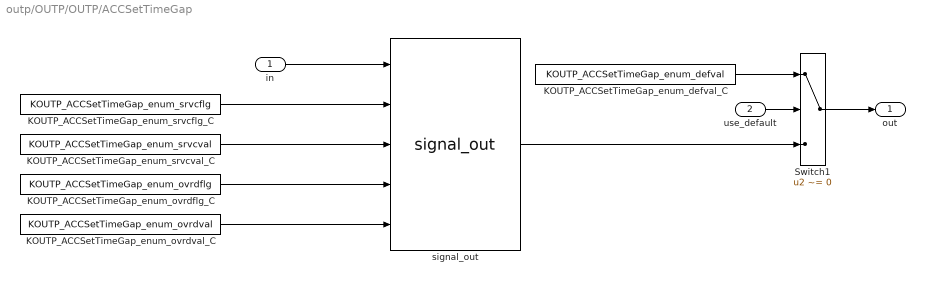
== system outp/OUTP/OUTP/ACCSetTimeGap ==
  in : Inport
  use_default : Inport  Port=2
  KOUTP_ACCSetTimeGap_enum_defval_C : Constant  Value=KOUTP_ACCSetTimeGap_enum_defval
  KOUTP_ACCSetTimeGap_enum_ovrdflg_C : Constant  Value=KOUTP_ACCSetTimeGap_enum_ovrdflg
  KOUTP_ACCSetTimeGap_enum_ovrdval_C : Constant  Value=KOUTP_ACCSetTimeGap_enum_ovrdval
  KOUTP_ACCSetTimeGap_enum_srvcflg_C : Constant  Value=KOUTP_ACCSetTimeGap_enum_srvcflg
  KOUTP_ACCSetTimeGap_enum_srvcval_C : Constant  Value=KOUTP_ACCSetTimeGap_enum_srvcval
  Switch1 : Switch  Criteria=u2 ~= 0  Threshold=0.5
  signal_out : outp/signal_out
  out : Outport
  wires:
  KOUTP_ACCSetTimeGap_enum_defval_C/1 -> Switch1/1
  KOUTP_ACCSetTimeGap_enum_ovrdval_C/1 -> signal_out/5
  KOUTP_ACCSetTimeGap_enum_ovrdflg_C/1 -> signal_out/4
  KOUTP_ACCSetTimeGap_enum_srvcval_C/1 -> signal_out/3
  KOUTP_ACCSetTimeGap_enum_srvcflg_C/1 -> signal_out/2
  Switch1/1 -> out/1
  use_default/1 -> Switch1/2
  signal_out/1 -> Switch1/3
  in/1 -> signal_out/1

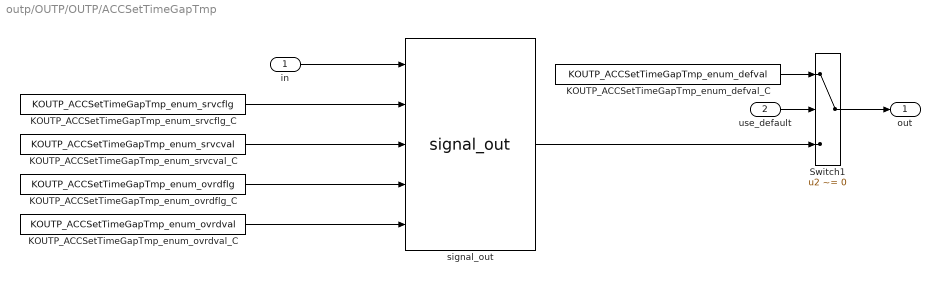
== system outp/OUTP/OUTP/ACCSetTimeGapTmp ==
  in : Inport
  use_default : Inport  Port=2
  KOUTP_ACCSetTimeGapTmp_enum_defval_C : Constant  Value=KOUTP_ACCSetTimeGapTmp_enum_defval
  KOUTP_ACCSetTimeGapTmp_enum_ovrdflg_C : Constant  Value=KOUTP_ACCSetTimeGapTmp_enum_ovrdflg
  KOUTP_ACCSetTimeGapTmp_enum_ovrdval_C : Constant  Value=KOUTP_ACCSetTimeGapTmp_enum_ovrdval
  KOUTP_ACCSetTimeGapTmp_enum_srvcflg_C : Constant  Value=KOUTP_ACCSetTimeGapTmp_enum_srvcflg
  KOUTP_ACCSetTimeGapTmp_enum_srvcval_C : Constant  Value=KOUTP_ACCSetTimeGapTmp_enum_srvcval
  Switch1 : Switch  Criteria=u2 ~= 0  Threshold=0.5
  signal_out : outp/signal_out
  out : Outport
  wires:
  in/1 -> signal_out/1
  signal_out/1 -> Switch1/3
  use_default/1 -> Switch1/2
  Switch1/1 -> out/1
  KOUTP_ACCSetTimeGapTmp_enum_srvcflg_C/1 -> signal_out/2
  KOUTP_ACCSetTimeGapTmp_enum_srvcval_C/1 -> signal_out/3
  KOUTP_ACCSetTimeGapTmp_enum_ovrdflg_C/1 -> signal_out/4
  KOUTP_ACCSetTimeGapTmp_enum_ovrdval_C/1 -> signal_out/5
  KOUTP_ACCSetTimeGapTmp_enum_defval_C/1 -> Switch1/1

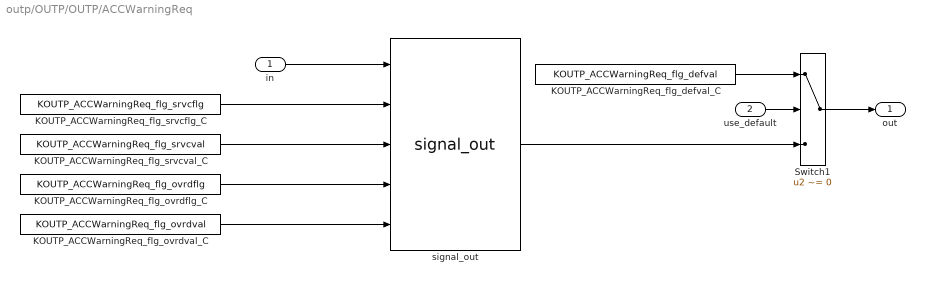
== system outp/OUTP/OUTP/ACCWarningReq ==
  in : Inport
  use_default : Inport  Port=2
  KOUTP_ACCWarningReq_flg_defval_C : Constant  Value=KOUTP_ACCWarningReq_flg_defval
  KOUTP_ACCWarningReq_flg_ovrdflg_C : Constant  Value=KOUTP_ACCWarningReq_flg_ovrdflg
  KOUTP_ACCWarningReq_flg_ovrdval_C : Constant  Value=KOUTP_ACCWarningReq_flg_ovrdval
  KOUTP_ACCWarningReq_flg_srvcflg_C : Constant  Value=KOUTP_ACCWarningReq_flg_srvcflg
  KOUTP_ACCWarningReq_flg_srvcval_C : Constant  Value=KOUTP_ACCWarningReq_flg_srvcval
  Switch1 : Switch  Criteria=u2 ~= 0  Threshold=0.5
  signal_out : outp/signal_out
  out : Outport
  wires:
  in/1 -> signal_out/1
  signal_out/1 -> Switch1/3
  use_default/1 -> Switch1/2
  Switch1/1 -> out/1
  KOUTP_ACCWarningReq_flg_srvcflg_C/1 -> signal_out/2
  KOUTP_ACCWarningReq_flg_srvcval_C/1 -> signal_out/3
  KOUTP_ACCWarningReq_flg_ovrdflg_C/1 -> signal_out/4
  KOUTP_ACCWarningReq_flg_ovrdval_C/1 -> signal_out/5
  KOUTP_ACCWarningReq_flg_defval_C/1 -> Switch1/1

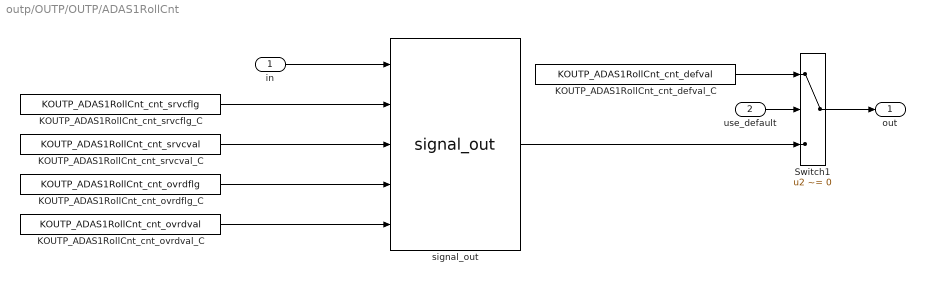
== system outp/OUTP/OUTP/ADAS1RollCnt ==
  in : Inport
  use_default : Inport  Port=2
  KOUTP_ADAS1RollCnt_cnt_defval_C : Constant  Value=KOUTP_ADAS1RollCnt_cnt_defval
  KOUTP_ADAS1RollCnt_cnt_ovrdflg_C : Constant  Value=KOUTP_ADAS1RollCnt_cnt_ovrdflg
  KOUTP_ADAS1RollCnt_cnt_ovrdval_C : Constant  Value=KOUTP_ADAS1RollCnt_cnt_ovrdval
  KOUTP_ADAS1RollCnt_cnt_srvcflg_C : Constant  Value=KOUTP_ADAS1RollCnt_cnt_srvcflg
  KOUTP_ADAS1RollCnt_cnt_srvcval_C : Constant  Value=KOUTP_ADAS1RollCnt_cnt_srvcval
  Switch1 : Switch  Criteria=u2 ~= 0  Threshold=0.5
  signal_out : outp/signal_out
  out : Outport
  wires:
  in/1 -> signal_out/1
  signal_out/1 -> Switch1/3
  use_default/1 -> Switch1/2
  Switch1/1 -> out/1
  KOUTP_ADAS1RollCnt_cnt_srvcflg_C/1 -> signal_out/2
  KOUTP_ADAS1RollCnt_cnt_srvcval_C/1 -> signal_out/3
  KOUTP_ADAS1RollCnt_cnt_ovrdflg_C/1 -> signal_out/4
  KOUTP_ADAS1RollCnt_cnt_ovrdval_C/1 -> signal_out/5
  KOUTP_ADAS1RollCnt_cnt_defval_C/1 -> Switch1/1

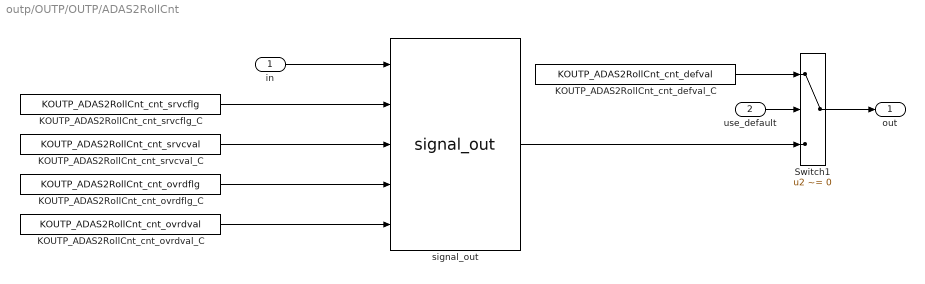
== system outp/OUTP/OUTP/ADAS2RollCnt ==
  in : Inport
  use_default : Inport  Port=2
  KOUTP_ADAS2RollCnt_cnt_defval_C : Constant  Value=KOUTP_ADAS2RollCnt_cnt_defval
  KOUTP_ADAS2RollCnt_cnt_ovrdflg_C : Constant  Value=KOUTP_ADAS2RollCnt_cnt_ovrdflg
  KOUTP_ADAS2RollCnt_cnt_ovrdval_C : Constant  Value=KOUTP_ADAS2RollCnt_cnt_ovrdval
  KOUTP_ADAS2RollCnt_cnt_srvcflg_C : Constant  Value=KOUTP_ADAS2RollCnt_cnt_srvcflg
  KOUTP_ADAS2RollCnt_cnt_srvcval_C : Constant  Value=KOUTP_ADAS2RollCnt_cnt_srvcval
  Switch1 : Switch  Criteria=u2 ~= 0  Threshold=0.5
  signal_out : outp/signal_out
  out : Outport
  wires:
  KOUTP_ADAS2RollCnt_cnt_defval_C/1 -> Switch1/1
  KOUTP_ADAS2RollCnt_cnt_ovrdval_C/1 -> signal_out/5
  KOUTP_ADAS2RollCnt_cnt_ovrdflg_C/1 -> signal_out/4
  KOUTP_ADAS2RollCnt_cnt_srvcval_C/1 -> signal_out/3
  KOUTP_ADAS2RollCnt_cnt_srvcflg_C/1 -> signal_out/2
  Switch1/1 -> out/1
  use_default/1 -> Switch1/2
  signal_out/1 -> Switch1/3
  in/1 -> signal_out/1

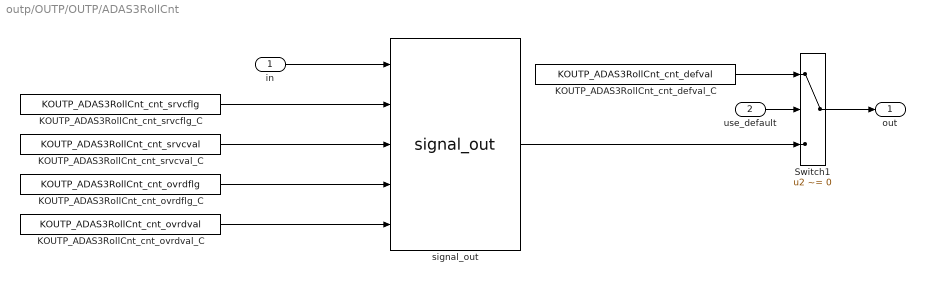
== system outp/OUTP/OUTP/ADAS3RollCnt ==
  in : Inport
  use_default : Inport  Port=2
  KOUTP_ADAS3RollCnt_cnt_defval_C : Constant  Value=KOUTP_ADAS3RollCnt_cnt_defval
  KOUTP_ADAS3RollCnt_cnt_ovrdflg_C : Constant  Value=KOUTP_ADAS3RollCnt_cnt_ovrdflg
  KOUTP_ADAS3RollCnt_cnt_ovrdval_C : Constant  Value=KOUTP_ADAS3RollCnt_cnt_ovrdval
  KOUTP_ADAS3RollCnt_cnt_srvcflg_C : Constant  Value=KOUTP_ADAS3RollCnt_cnt_srvcflg
  KOUTP_ADAS3RollCnt_cnt_srvcval_C : Constant  Value=KOUTP_ADAS3RollCnt_cnt_srvcval
  Switch1 : Switch  Criteria=u2 ~= 0  Threshold=0.5
  signal_out : outp/signal_out
  out : Outport
  wires:
  in/1 -> signal_out/1
  signal_out/1 -> Switch1/3
  use_default/1 -> Switch1/2
  Switch1/1 -> out/1
  KOUTP_ADAS3RollCnt_cnt_srvcflg_C/1 -> signal_out/2
  KOUTP_ADAS3RollCnt_cnt_srvcval_C/1 -> signal_out/3
  KOUTP_ADAS3RollCnt_cnt_ovrdflg_C/1 -> signal_out/4
  KOUTP_ADAS3RollCnt_cnt_ovrdval_C/1 -> signal_out/5
  KOUTP_ADAS3RollCnt_cnt_defval_C/1 -> Switch1/1

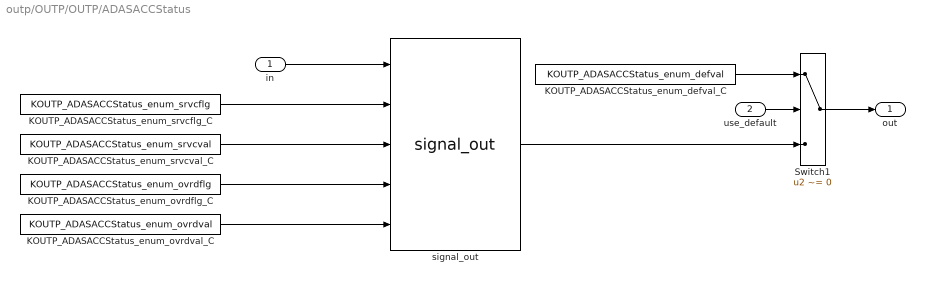
== system outp/OUTP/OUTP/ADASACCStatus ==
  in : Inport
  use_default : Inport  Port=2
  KOUTP_ADASACCStatus_enum_defval_C : Constant  Value=KOUTP_ADASACCStatus_enum_defval
  KOUTP_ADASACCStatus_enum_ovrdflg_C : Constant  Value=KOUTP_ADASACCStatus_enum_ovrdflg
  KOUTP_ADASACCStatus_enum_ovrdval_C : Constant  Value=KOUTP_ADASACCStatus_enum_ovrdval
  KOUTP_ADASACCStatus_enum_srvcflg_C : Constant  Value=KOUTP_ADASACCStatus_enum_srvcflg
  KOUTP_ADASACCStatus_enum_srvcval_C : Constant  Value=KOUTP_ADASACCStatus_enum_srvcval
  Switch1 : Switch  Criteria=u2 ~= 0  Threshold=0.5
  signal_out : outp/signal_out
  out : Outport
  wires:
  in/1 -> signal_out/1
  signal_out/1 -> Switch1/3
  use_default/1 -> Switch1/2
  Switch1/1 -> out/1
  KOUTP_ADASACCStatus_enum_srvcflg_C/1 -> signal_out/2
  KOUTP_ADASACCStatus_enum_srvcval_C/1 -> signal_out/3
  KOUTP_ADASACCStatus_enum_ovrdflg_C/1 -> signal_out/4
  KOUTP_ADASACCStatus_enum_ovrdval_C/1 -> signal_out/5
  KOUTP_ADASACCStatus_enum_defval_C/1 -> Switch1/1

== system outp/OUTP/OUTP/ADASFaultMode ==
  in : Inport
  use_default : Inport  Port=2
  KOUTP_ADASFaultMode_enum_defval_C : Constant  Value=KOUTP_ADASFaultMode_enum_defval
  KOUTP_ADASFaultMode_enum_ovrdflg_C : Constant  Value=KOUTP_ADASFaultMode_enum_ovrdflg
  KOUTP_ADASFaultMode_enum_ovrdval_C : Constant  Value=KOUTP_ADASFaultMode_enum_ovrdval
  KOUTP_ADASFaultMode_enum_srvcflg_C : Constant  Value=KOUTP_ADASFaultMode_enum_srvcflg
  KOUTP_ADASFaultMode_enum_srvcval_C : Constant  Value=KOUTP_ADASFaultMode_enum_srvcval
  Switch1 : Switch  Criteria=u2 ~= 0  Threshold=0.5
  signal_out : outp/signal_out
  out : Outport
  wires:
  in/1 -> signal_out/1
  signal_out/1 -> Switch1/3
  use_default/1 -> Switch1/2
  Switch1/1 -> out/1
  KOUTP_ADASFaultMode_enum_srvcflg_C/1 -> signal_out/2
  KOUTP_ADASFaultMode_enum_srvcval_C/1 -> signal_out/3
  KOUTP_ADASFaultMode_enum_ovrdflg_C/1 -> signal_out/4
  KOUTP_ADASFaultMode_enum_ovrdval_C/1 -> signal_out/5
  KOUTP_ADASFaultMode_enum_defval_C/1 -> Switch1/1
